simulink model "Q6"  (R2015a)
settings: Solver=ode45  StartTime=0.0  StopTime=10.0  RelTol=1e-3
values from neighbouring files (symbols this model uses):
  C1 = eye(5)    [LabCEE.m]
  D1 = [0 0 0 0 0;0 0 0 0 0]'    [LabCEE.m]
  K = lqr(A, B, Qr, Rr)    [LabCEE.m]    (also in fp_ini.m; test.m)
  x_0 = [0.1 0 0 0 0]'    [LabCEE.m]    (also in test.m)
undefined symbols (not defined in the file or in its folder): A, B
settings Model: Creator=Alunos  LastModifiedBy=Alunos

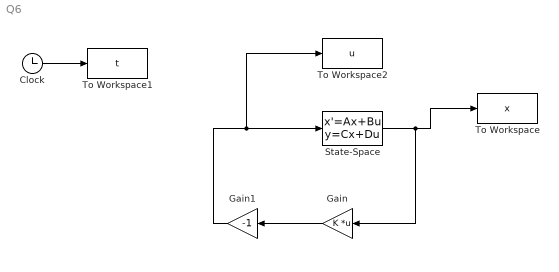
== system Q6 ==
  Clock : Clock
  Gain : Gain  Gain=K  Multiplication=Matrix(K*u)
  Gain1 : Gain  Gain=-1
  State-Space : StateSpace  A=A  B=B  C=C1  D=D1  X0=x_0
  To Workspace : ToWorkspace  VariableName=x  SampleTime=-1
  To Workspace1 : ToWorkspace  VariableName=t  SampleTime=-1
  To Workspace2 : ToWorkspace  VariableName=u  SampleTime=-1
  wires:
  Clock/1 -> To Workspace1/1
  State-Space/1 -> Gain/1, To Workspace/1
  Gain/1 -> Gain1/1
  Gain1/1 -> To Workspace2/1, State-Space/1
